simulink model "MyPTControl_RTW"  (Simulink 7.5)
settings: Solver=ode1  SolverMode=SingleTasking  StartTime=0.0  StopTime=inf  FixedStep=0.0002  RelTol=1e-3
PreLoadFcn:
  | vehicle = 'Car'; if ~length(which('cmcmd')), cmenv; end
  | MyPTControl_RTW_bus
InitFcn:
  | vehicle = 'Car'; if ~length(which('cmcmd')), cmenv; end
  | MyPTControl_RTW_bus
undefined symbols (not defined in the file or in its folder): EngineOut_Load, EngineOut_set_ISC, Ignition, ISGOut_Load, OperationState
libraries: simulink x11
Description:
  | CarMaker Real-Time Target (generic)
settings Model: Creator=ml  LastModifiedBy=ml
settings DebuggingCC: SolverPrmCheckMsg=none
settings HardwareCC: TargetHWDeviceType=32-bit Generic  ProdEqTarget=off
settings RTWCC: SystemTargetFile=CarMaker.tlc  TemplateMakefile=CarMaker_unix.tmf  Description=CarMaker Real-Time Target (32-bit)  ProcessScript=CarMaker_make_rtw_hook
settings CodeAppCC: MaxIdLength=63
settings STFCustomTargetCC: ModelReferenceCompliant=off  GeneratePreprocessorConditionals=Disable all  SystemTargetFile=CarMaker.tlc
settings GRTTargetCC: ModelReferenceCompliant=off  ParMdlRefBuildCompliant=off  CompOptLevelCompliant=off  MatFileLogging=off  ExtModeMexFile=noextcomm
settings CustomProperty: DataType=string  Value=..
settings EnumStrPairs: String=Car

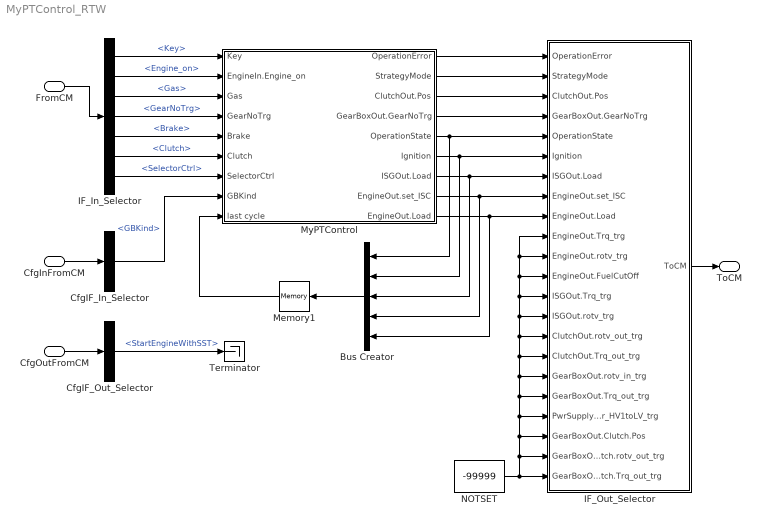
== system MyPTControl_RTW ==
  FromCM : Inport  UseBusObject=on
      settings: BusObject=cmPTControlIn
  CfgInFromCM : Inport  Port=2  UseBusObject=on
      settings: BusObject=cmPTControlCfgIn
  CfgOutFromCM : Inport  Port=3  UseBusObject=on
      settings: BusObject=cmPTControlCfgOut
  Bus Creator : BusCreator  Inputs=5
  CfgIF_In_Selector : BusSelector  OutputSignals=GearBox.GBKind
  CfgIF_Out_Selector : BusSelector  OutputSignals=StartEngineWithSST
  IF_In_Selector : BusSelector  OutputSignals=Key,EngineIn.Engine_on,Gas,GearNoTrg,Brake,Clutch,SelectorCtrl
  IF_Out_Selector : Subsystem
      settings: OpenFcn=cmSignalSelect('SignalSelection_CB',gcb)
      mask Type: Signal Selection
      mask Description: Signal Selection Block
  Memory1 : Memory
  MyPTControl : Subsystem
  NOTSET : Constant  Value=-99999  OutDataType=sfix(16)  OutScaling=2^0
  Terminator : Terminator
  ToCM : Outport  UseBusObject=on
      settings: BusObject=cmPTControlOut
  wires:
  FromCM/1 -> IF_In_Selector/1
  IF_Out_Selector/1(ToCM) -> ToCM/1
  Bus Creator/1 -> Memory1/1
  Memory1/1 -> MyPTControl/9(last cycle)
  MyPTControl/5(OperationState) -> Bus Creator/1, IF_Out_Selector/5(OperationState)
  MyPTControl/6(Ignition) -> Bus Creator/2, IF_Out_Selector/6(Ignition)
  MyPTControl/7(ISGOut.Load) -> Bus Creator/3, IF_Out_Selector/7(ISGOut.Load)
  MyPTControl/8(EngineOut.set_ISC) -> Bus Creator/4, IF_Out_Selector/8(EngineOut.set_ISC)
  MyPTControl/9(EngineOut.Load) -> Bus Creator/5, IF_Out_Selector/9(EngineOut.Load)
  MyPTControl/1(OperationError) -> IF_Out_Selector/1(OperationError)
  MyPTControl/2(StrategyMode) -> IF_Out_Selector/2(StrategyMode)
  MyPTControl/3(ClutchOut.Pos) -> IF_Out_Selector/3(ClutchOut.Pos)
  MyPTControl/4(GearBoxOut.GearNoTrg) -> IF_Out_Selector/4(GearBoxOut.GearNoTrg)
  NOTSET/1 -> IF_Out_Selector/21(GearBoxOut.Clutch.rotv_out_trg), IF_Out_Selector/22(GearBoxOut.Clutch.Trq_out_trg), IF_Out_Selector/20(GearBoxOut.Clutch.Pos), IF_Out_Selector/19(PwrSupplyOut.Pwr_HV1toLV_trg), IF_Out_Selector/11(EngineOut.rotv_trg), IF_Out_Selector/10(EngineOut.Trq_trg), IF_Out_Selector/12(EngineOut.FuelCutOff), IF_Out_Selector/13(ISGOut.Trq_trg), IF_Out_Selector/14(ISGOut.rotv_trg), IF_Out_Selector/15(ClutchOut.rotv_out_trg), IF_Out_Selector/16(ClutchOut.Trq_out_trg), IF_Out_Selector/17(GearBoxOut.rotv_in_trg), IF_Out_Selector/18(GearBoxOut.Trq_out_trg)
  IF_In_Selector/1 -> MyPTControl/1(Key)  "<Key>"
  IF_In_Selector/2 -> MyPTControl/2(EngineIn.Engine_on)  "<Engine_on>"
  IF_In_Selector/3 -> MyPTControl/3(Gas)  "<Gas>"
  IF_In_Selector/4 -> MyPTControl/4(GearNoTrg)  "<GearNoTrg>"
  IF_In_Selector/5 -> MyPTControl/5(Brake)  "<Brake>"
  IF_In_Selector/6 -> MyPTControl/6(Clutch)  "<Clutch>"
  IF_In_Selector/7 -> MyPTControl/7(SelectorCtrl)  "<SelectorCtrl>"
  CfgInFromCM/1 -> CfgIF_In_Selector/1
  CfgOutFromCM/1 -> CfgIF_Out_Selector/1
  CfgIF_In_Selector/1 -> MyPTControl/8(GBKind)  "<GBKind>"
  CfgIF_Out_Selector/1 -> Terminator/1  "<StartEngineWithSST>"

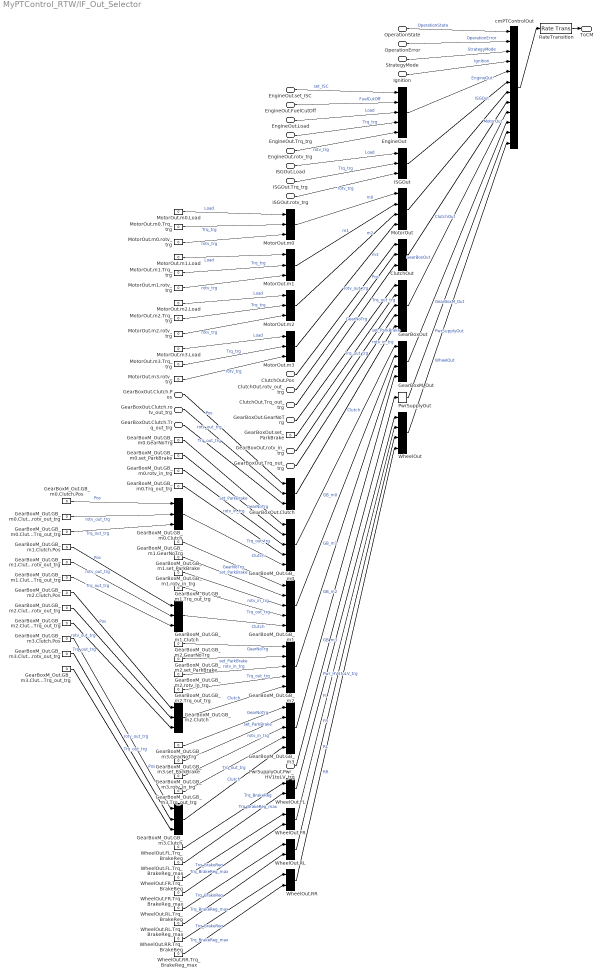
== system MyPTControl_RTW/IF_Out_Selector ==
  OperationError : Inport
  StrategyMode : Inport  Port=2
  ClutchOut.Pos : Inport  Port=3
  GearBoxOut.GearNoTrg : Inport  Port=4
  OperationState : Inport  Port=5
  Ignition : Inport  Port=6
  ISGOut.Load : Inport  Port=7
  EngineOut.set_ISC : Inport  Port=8
  EngineOut.Load : Inport  Port=9
  EngineOut.Trq_trg : Inport  Port=10
  EngineOut.rotv_trg : Inport  Port=11
  EngineOut.FuelCutOff : Inport  Port=12
  ISGOut.Trq_trg : Inport  Port=13
  ISGOut.rotv_trg : Inport  Port=14
  ClutchOut.rotv_out_trg : Inport  Port=15
  ClutchOut.Trq_out_trg : Inport  Port=16
  GearBoxOut.rotv_in_trg : Inport  Port=17
  GearBoxOut.Trq_out_trg : Inport  Port=18
  PwrSupplyOut.Pwr_HV1toLV_trg : Inport  Port=19
  GearBoxOut.Clutch.Pos : Inport  Port=20
  GearBoxOut.Clutch.rotv_out_trg : Inport  Port=21
  GearBoxOut.Clutch.Trq_out_trg : Inport  Port=22
  ClutchOut : BusCreator  Inputs=3
  EngineOut : BusCreator  Inputs=5
  GearBoxM_Out : BusCreator
  GearBoxM_Out.GB_m{0..3} (4 alike) : BusCreator  Inputs=5
  GearBoxM_Out.GB_m0.Clutch : BusCreator  Inputs=3
  GearBoxM_Out.GB_m0.Clutch.Pos : Constant  Value=0
  GearBoxM_Out.GB_m0.Clutch.Trq_out_trg : Constant  Value=0
  GearBoxM_Out.GB_m0.Clutch.rotv_out_trg : Constant  Value=0
  GearBoxM_Out.GB_m0.GearNoTrg : Constant  Value=0
  GearBoxM_Out.GB_m0.Trq_out_trg : Constant  Value=0
  GearBoxM_Out.GB_m0.rotv_in_trg : Constant  Value=0
  GearBoxM_Out.GB_m0.set_ParkBrake : Constant  Value=0
  GearBoxM_Out.GB_m1.Clutch : BusCreator  Inputs=3
  GearBoxM_Out.GB_m1.Clutch.Pos : Constant  Value=0
  GearBoxM_Out.GB_m1.Clutch.Trq_out_trg : Constant  Value=0
  GearBoxM_Out.GB_m1.Clutch.rotv_out_trg : Constant  Value=0
  GearBoxM_Out.GB_m1.GearNoTrg : Constant  Value=0
  GearBoxM_Out.GB_m1.Trq_out_trg : Constant  Value=0
  GearBoxM_Out.GB_m1.rotv_in_trg : Constant  Value=0
  GearBoxM_Out.GB_m1.set_ParkBrake : Constant  Value=0
  GearBoxM_Out.GB_m2.Clutch : BusCreator  Inputs=3
  GearBoxM_Out.GB_m2.Clutch.Pos : Constant  Value=0
  GearBoxM_Out.GB_m2.Clutch.Trq_out_trg : Constant  Value=0
  GearBoxM_Out.GB_m2.Clutch.rotv_out_trg : Constant  Value=0
  GearBoxM_Out.GB_m2.GearNoTrg : Constant  Value=0
  GearBoxM_Out.GB_m2.Trq_out_trg : Constant  Value=0
  GearBoxM_Out.GB_m2.rotv_in_trg : Constant  Value=0
  GearBoxM_Out.GB_m2.set_ParkBrake : Constant  Value=0
  GearBoxM_Out.GB_m3.Clutch : BusCreator  Inputs=3
  GearBoxM_Out.GB_m3.Clutch.Pos : Constant  Value=0
  GearBoxM_Out.GB_m3.Clutch.Trq_out_trg : Constant  Value=0
  GearBoxM_Out.GB_m3.Clutch.rotv_out_trg : Constant  Value=0
  GearBoxM_Out.GB_m3.GearNoTrg : Constant  Value=0
  GearBoxM_Out.GB_m3.Trq_out_trg : Constant  Value=0
  GearBoxM_Out.GB_m3.rotv_in_trg : Constant  Value=0
  GearBoxM_Out.GB_m3.set_ParkBrake : Constant  Value=0
  GearBoxOut : BusCreator  Inputs=5
  GearBoxOut.Clutch : BusCreator  Inputs=3
  GearBoxOut.set_ParkBrake : Constant  Value=0
  ISGOut : BusCreator  Inputs=3
  MotorOut : BusCreator
  MotorOut.m{0..3} (4 alike) : BusCreator  Inputs=3
  MotorOut.m0.Load : Constant  Value=0
  MotorOut.m0.Trq_trg : Constant  Value=0
  MotorOut.m0.rotv_trg : Constant  Value=0
  MotorOut.m1.Load : Constant  Value=0
  MotorOut.m1.Trq_trg : Constant  Value=0
  MotorOut.m1.rotv_trg : Constant  Value=0
  MotorOut.m2.Load : Constant  Value=0
  MotorOut.m2.Trq_trg : Constant  Value=0
  MotorOut.m2.rotv_trg : Constant  Value=0
  MotorOut.m3.Load : Constant  Value=0
  MotorOut.m3.Trq_trg : Constant  Value=0
  MotorOut.m3.rotv_trg : Constant  Value=0
  PwrSupplyOut : BusCreator  Inputs=1
  RateTransition : RateTransition  OutPortSampleTime=str2num(get_param(gcs,'FixedStep'))
  WheelOut : BusCreator
  WheelOut.FL : BusCreator  Inputs=2
  WheelOut.FL.Trq_BrakeReg : Constant  Value=0
  WheelOut.FL.Trq_BrakeReg_max : Constant  Value=0
  WheelOut.FR : BusCreator  Inputs=2
  WheelOut.FR.Trq_BrakeReg : Constant  Value=0
  WheelOut.FR.Trq_BrakeReg_max : Constant  Value=0
  WheelOut.RL : BusCreator  Inputs=2
  WheelOut.RL.Trq_BrakeReg : Constant  Value=0
  WheelOut.RL.Trq_BrakeReg_max : Constant  Value=0
  WheelOut.RR : BusCreator  Inputs=2
  WheelOut.RR.Trq_BrakeReg : Constant  Value=0
  WheelOut.RR.Trq_BrakeReg_max : Constant  Value=0
  cmPTControlOut : BusCreator  Inputs=12
  ToCM : Outport
  wires:
  RateTransition/1 -> ToCM/1
  cmPTControlOut/1 -> RateTransition/1
  EngineOut/1 -> cmPTControlOut/5  "EngineOut"
  ISGOut/1 -> cmPTControlOut/6  "ISGOut"
  MotorOut/1 -> cmPTControlOut/7  "MotorOut"
  MotorOut.m0/1 -> MotorOut/1  "m0"
  MotorOut.m0.Load/1 -> MotorOut.m0/1  "Load"
  MotorOut.m0.Trq_trg/1 -> MotorOut.m0/2  "Trq_trg"
  MotorOut.m0.rotv_trg/1 -> MotorOut.m0/3  "rotv_trg"
  MotorOut.m1/1 -> MotorOut/2  "m1"
  MotorOut.m1.Load/1 -> MotorOut.m1/1  "Load"
  MotorOut.m1.Trq_trg/1 -> MotorOut.m1/2  "Trq_trg"
  MotorOut.m1.rotv_trg/1 -> MotorOut.m1/3  "rotv_trg"
  MotorOut.m2/1 -> MotorOut/3  "m2"
  MotorOut.m2.Load/1 -> MotorOut.m2/1  "Load"
  MotorOut.m2.Trq_trg/1 -> MotorOut.m2/2  "Trq_trg"
  MotorOut.m2.rotv_trg/1 -> MotorOut.m2/3  "rotv_trg"
  MotorOut.m3/1 -> MotorOut/4  "m3"
  MotorOut.m3.Load/1 -> MotorOut.m3/1  "Load"
  MotorOut.m3.Trq_trg/1 -> MotorOut.m3/2  "Trq_trg"
  MotorOut.m3.rotv_trg/1 -> MotorOut.m3/3  "rotv_trg"
  ClutchOut/1 -> cmPTControlOut/8  "ClutchOut"
  GearBoxOut/1 -> cmPTControlOut/9  "GearBoxOut"
  GearBoxOut.set_ParkBrake/1 -> GearBoxOut/2  "set_ParkBrake"
  GearBoxOut.Clutch/1 -> GearBoxOut/5  "Clutch"
  GearBoxM_Out/1 -> cmPTControlOut/10  "GearBoxM_Out"
  GearBoxM_Out.GB_m0/1 -> GearBoxM_Out/1  "GB_m0"
  GearBoxM_Out.GB_m0.GearNoTrg/1 -> GearBoxM_Out.GB_m0/1  "GearNoTrg"
  GearBoxM_Out.GB_m0.set_ParkBrake/1 -> GearBoxM_Out.GB_m0/2  "set_ParkBrake"
  GearBoxM_Out.GB_m0.rotv_in_trg/1 -> GearBoxM_Out.GB_m0/3  "rotv_in_trg"
  GearBoxM_Out.GB_m0.Trq_out_trg/1 -> GearBoxM_Out.GB_m0/4  "Trq_out_trg"
  GearBoxM_Out.GB_m0.Clutch/1 -> GearBoxM_Out.GB_m0/5  "Clutch"
  GearBoxM_Out.GB_m0.Clutch.Pos/1 -> GearBoxM_Out.GB_m0.Clutch/1  "Pos"
  GearBoxM_Out.GB_m0.Clutch.rotv_out_trg/1 -> GearBoxM_Out.GB_m0.Clutch/2  "rotv_out_trg"
  GearBoxM_Out.GB_m0.Clutch.Trq_out_trg/1 -> GearBoxM_Out.GB_m0.Clutch/3  "Trq_out_trg"
  GearBoxM_Out.GB_m1/1 -> GearBoxM_Out/2  "GB_m1"
  GearBoxM_Out.GB_m1.GearNoTrg/1 -> GearBoxM_Out.GB_m1/1  "GearNoTrg"
  GearBoxM_Out.GB_m1.set_ParkBrake/1 -> GearBoxM_Out.GB_m1/2  "set_ParkBrake"
  GearBoxM_Out.GB_m1.rotv_in_trg/1 -> GearBoxM_Out.GB_m1/3  "rotv_in_trg"
  GearBoxM_Out.GB_m1.Trq_out_trg/1 -> GearBoxM_Out.GB_m1/4  "Trq_out_trg"
  GearBoxM_Out.GB_m1.Clutch/1 -> GearBoxM_Out.GB_m1/5  "Clutch"
  GearBoxM_Out.GB_m1.Clutch.Pos/1 -> GearBoxM_Out.GB_m1.Clutch/1  "Pos"
  GearBoxM_Out.GB_m1.Clutch.rotv_out_trg/1 -> GearBoxM_Out.GB_m1.Clutch/2  "rotv_out_trg"
  GearBoxM_Out.GB_m1.Clutch.Trq_out_trg/1 -> GearBoxM_Out.GB_m1.Clutch/3  "Trq_out_trg"
  GearBoxM_Out.GB_m2/1 -> GearBoxM_Out/3  "GB_m2"
  GearBoxM_Out.GB_m2.GearNoTrg/1 -> GearBoxM_Out.GB_m2/1  "GearNoTrg"
  GearBoxM_Out.GB_m2.set_ParkBrake/1 -> GearBoxM_Out.GB_m2/2  "set_ParkBrake"
  GearBoxM_Out.GB_m2.rotv_in_trg/1 -> GearBoxM_Out.GB_m2/3  "rotv_in_trg"
  GearBoxM_Out.GB_m2.Trq_out_trg/1 -> GearBoxM_Out.GB_m2/4  "Trq_out_trg"
  GearBoxM_Out.GB_m2.Clutch/1 -> GearBoxM_Out.GB_m2/5  "Clutch"
  GearBoxM_Out.GB_m2.Clutch.Pos/1 -> GearBoxM_Out.GB_m2.Clutch/1  "Pos"
  GearBoxM_Out.GB_m2.Clutch.rotv_out_trg/1 -> GearBoxM_Out.GB_m2.Clutch/2  "rotv_out_trg"
  GearBoxM_Out.GB_m2.Clutch.Trq_out_trg/1 -> GearBoxM_Out.GB_m2.Clutch/3  "Trq_out_trg"
  GearBoxM_Out.GB_m3/1 -> GearBoxM_Out/4  "GB_m3"
  GearBoxM_Out.GB_m3.GearNoTrg/1 -> GearBoxM_Out.GB_m3/1  "GearNoTrg"
  GearBoxM_Out.GB_m3.set_ParkBrake/1 -> GearBoxM_Out.GB_m3/2  "set_ParkBrake"
  GearBoxM_Out.GB_m3.rotv_in_trg/1 -> GearBoxM_Out.GB_m3/3  "rotv_in_trg"
  GearBoxM_Out.GB_m3.Trq_out_trg/1 -> GearBoxM_Out.GB_m3/4  "Trq_out_trg"
  GearBoxM_Out.GB_m3.Clutch/1 -> GearBoxM_Out.GB_m3/5  "Clutch"
  GearBoxM_Out.GB_m3.Clutch.Pos/1 -> GearBoxM_Out.GB_m3.Clutch/1  "Pos"
  GearBoxM_Out.GB_m3.Clutch.rotv_out_trg/1 -> GearBoxM_Out.GB_m3.Clutch/2  "rotv_out_trg"
  GearBoxM_Out.GB_m3.Clutch.Trq_out_trg/1 -> GearBoxM_Out.GB_m3.Clutch/3  "Trq_out_trg"
  PwrSupplyOut/1 -> cmPTControlOut/11  "PwrSupplyOut"
  WheelOut/1 -> cmPTControlOut/12  "WheelOut"
  WheelOut.FL/1 -> WheelOut/1  "FL"
  WheelOut.FL.Trq_BrakeReg/1 -> WheelOut.FL/1  "Trq_BrakeReg"
  WheelOut.FL.Trq_BrakeReg_max/1 -> WheelOut.FL/2  "Trq_BrakeReg_max"
  WheelOut.FR/1 -> WheelOut/2  "FR"
  WheelOut.FR.Trq_BrakeReg/1 -> WheelOut.FR/1  "Trq_BrakeReg"
  WheelOut.FR.Trq_BrakeReg_max/1 -> WheelOut.FR/2  "Trq_BrakeReg_max"
  WheelOut.RL/1 -> WheelOut/3  "RL"
  WheelOut.RL.Trq_BrakeReg/1 -> WheelOut.RL/1  "Trq_BrakeReg"
  WheelOut.RL.Trq_BrakeReg_max/1 -> WheelOut.RL/2  "Trq_BrakeReg_max"
  WheelOut.RR/1 -> WheelOut/4  "RR"
  WheelOut.RR.Trq_BrakeReg/1 -> WheelOut.RR/1  "Trq_BrakeReg"
  WheelOut.RR.Trq_BrakeReg_max/1 -> WheelOut.RR/2  "Trq_BrakeReg_max"
  OperationError/1 -> cmPTControlOut/2  "OperationError"
  StrategyMode/1 -> cmPTControlOut/3  "StrategyMode"
  ClutchOut.Pos/1 -> ClutchOut/1  "Pos"
  GearBoxOut.GearNoTrg/1 -> GearBoxOut/1  "GearNoTrg"
  OperationState/1 -> cmPTControlOut/1  "OperationState"
  Ignition/1 -> cmPTControlOut/4  "Ignition"
  ISGOut.Load/1 -> ISGOut/1  "Load"
  EngineOut.set_ISC/1 -> EngineOut/1  "set_ISC"
  EngineOut.Load/1 -> EngineOut/3  "Load"
  EngineOut.Trq_trg/1 -> EngineOut/4  "Trq_trg"
  EngineOut.rotv_trg/1 -> EngineOut/5  "rotv_trg"
  EngineOut.FuelCutOff/1 -> EngineOut/2  "FuelCutOff"
  ISGOut.Trq_trg/1 -> ISGOut/2  "Trq_trg"
  ISGOut.rotv_trg/1 -> ISGOut/3  "rotv_trg"
  ClutchOut.rotv_out_trg/1 -> ClutchOut/2  "rotv_out_trg"
  ClutchOut.Trq_out_trg/1 -> ClutchOut/3  "Trq_out_trg"
  GearBoxOut.rotv_in_trg/1 -> GearBoxOut/3  "rotv_in_trg"
  GearBoxOut.Trq_out_trg/1 -> GearBoxOut/4  "Trq_out_trg"
  PwrSupplyOut.Pwr_HV1toLV_trg/1 -> PwrSupplyOut/1  "Pwr_HV1toLV_trg"
  GearBoxOut.Clutch.Pos/1 -> GearBoxOut.Clutch/1  "Pos"
  GearBoxOut.Clutch.rotv_out_trg/1 -> GearBoxOut.Clutch/2  "rotv_out_trg"
  GearBoxOut.Clutch.Trq_out_trg/1 -> GearBoxOut.Clutch/3  "Trq_out_trg"

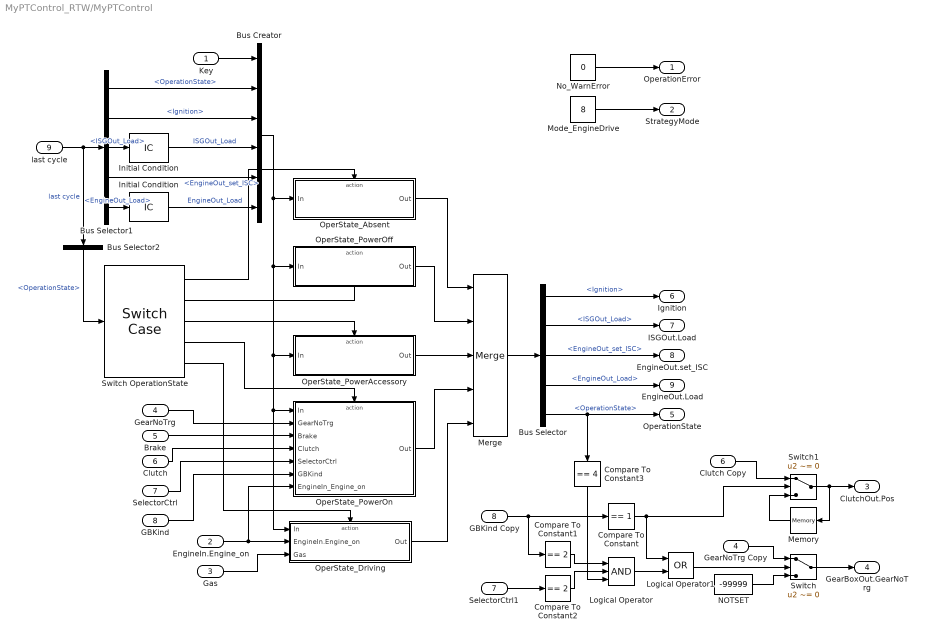
== system MyPTControl_RTW/MyPTControl ==
  Key : Inport  OutDataType=sfix(16)  OutScaling=2^0
  EngineIn.Engine_on : Inport  Port=2  OutDataType=sfix(16)  OutScaling=2^0
  Gas : Inport  Port=3  OutDataType=sfix(16)  OutScaling=2^0
  GearNoTrg : Inport  Port=4  OutDataType=sfix(16)  OutScaling=2^0
  Brake : Inport  Port=5  OutDataType=sfix(16)  OutScaling=2^0
  Clutch : Inport  Port=6  OutDataType=sfix(16)  OutScaling=2^0
  SelectorCtrl : Inport  Port=7  OutDataType=sfix(16)  OutScaling=2^0
  GBKind : Inport  Port=8  OutDataType=sfix(16)  OutScaling=2^0
  last cycle : Inport  Port=9  OutDataType=sfix(16)  OutScaling=2^0
  Bus Creator : BusCreator  Inputs=6
  Bus Selector : BusSelector  OutputSignals=Ignition,ISGOut_Load,EngineOut_set_ISC,EngineOut_Load,OperationState
  Bus Selector1 : BusSelector  OutputSignals=OperationState,Ignition,ISGOut_Load,EngineOut_set_ISC,EngineOut_Load
  Bus Selector2 : BusSelector  OutputSignals=OperationState
  Clutch Copy : InportShadow  Port=6  OutDataType=sfix(16)  OutScaling=2^0
  Compare To Constant : simulink/Logic and Bit Operations/Compare To Constant  SystemSampleTime=-1  relop===  const=1  LogicOutDataTypeMode=uint8  ZeroCross=off
  Compare To Constant1 : simulink/Logic and Bit Operations/Compare To Constant  SystemSampleTime=-1  relop===  const=2  LogicOutDataTypeMode=uint8  ZeroCross=off
  Compare To Constant2 : simulink/Logic and Bit Operations/Compare To Constant  SystemSampleTime=-1  relop===  const=2  LogicOutDataTypeMode=uint8  ZeroCross=off
  Compare To Constant3 : simulink/Logic and Bit Operations/Compare To Constant  SystemSampleTime=-1  relop===  const=4  LogicOutDataTypeMode=uint8  ZeroCross=off
  GBKind Copy : InportShadow  Port=8  OutDataType=sfix(16)  OutScaling=2^0
  GearNoTrg Copy : InportShadow  Port=4  OutDataType=sfix(16)  OutScaling=2^0
  Initial Condition : InitialCondition  Value=-99999
  "Initial Condition " : InitialCondition  Value=-99999
  Logical Operator : Logic  Inputs=3  AllPortsSameDT=off  OutDataTypeMode=boolean  OutDataTypeStr=boolean
  Logical Operator1 : Logic  Operator=OR  AllPortsSameDT=off  OutDataTypeMode=boolean  OutDataTypeStr=boolean
  Memory : Memory
  Merge : Merge  Inputs=5
  Mode_EngineDrive : Constant  Value=8  OutDataType=sfix(16)  OutScaling=2^0
  NOTSET : Constant  Value=-99999  OutDataType=sfix(16)  OutScaling=2^0
  No_WarnError : Constant  Value=0  OutDataType=sfix(16)  OutScaling=2^0
  OperState_Absent : Subsystem  TreatAsAtomicUnit=on
  OperState_Driving : Subsystem  TreatAsAtomicUnit=on
  OperState_PowerAccessory : Subsystem  TreatAsAtomicUnit=on
  OperState_PowerOff : Subsystem  TreatAsAtomicUnit=on
  OperState_PowerOn : Subsystem  TreatAsAtomicUnit=on
  SelectorCtrl1 : InportShadow  Port=7  OutDataType=sfix(16)  OutScaling=2^0
  Switch : Switch  Criteria=u2 ~= 0  OutDataType=sfix(16)  OutScaling=2^0
  Switch OperationState : SwitchCase  CaseConditions={0 1 2 3}
  Switch1 : Switch  Criteria=u2 ~= 0  OutDataType=sfix(16)  OutScaling=2^0
  OperationError : Outport  OutDataType=sfix(16)  OutScaling=2^0
  StrategyMode : Outport  Port=2  OutDataType=sfix(16)  OutScaling=2^0
  ClutchOut.Pos : Outport  Port=3  OutDataType=sfix(16)  OutScaling=2^0
  GearBoxOut.GearNoTrg : Outport  Port=4  OutDataType=sfix(16)  OutScaling=2^0
  OperationState : Outport  Port=5  OutDataType=sfix(16)  OutScaling=2^0
  Ignition : Outport  Port=6  OutDataType=sfix(16)  OutScaling=2^0
  ISGOut.Load : Outport  Port=7  OutDataType=sfix(16)  OutScaling=2^0
  EngineOut.set_ISC : Outport  Port=8  OutDataType=sfix(16)  OutScaling=2^0
  EngineOut.Load : Outport  Port=9  OutDataType=sfix(16)  OutScaling=2^0
  wires:
  No_WarnError/1 -> OperationError/1
  Mode_EngineDrive/1 -> StrategyMode/1
  Switch OperationState/3 -> OperState_PowerAccessory/Action
  Bus Selector/1 -> Ignition/1  "<Ignition>"
  Bus Selector/5 -> OperationState/1, Compare To Constant3/1  "<OperationState>"
  EngineIn.Engine_on/1 -> OperState_PowerOn/7(EngineIn_Engine_on), OperState_Driving/2(EngineIn.Engine_on)
  last cycle/1 -> Bus Selector2/1, Bus Selector1/1  "last cycle"
  Bus Selector2/1 -> Switch OperationState/1  "<OperationState>"
  Key/1 -> Bus Creator/1
  Bus Creator/1 -> OperState_Absent/1(In), OperState_PowerOff/1(In), OperState_PowerAccessory/1(In), OperState_PowerOn/1(In), OperState_Driving/1(In)
  Bus Selector/2 -> ISGOut.Load/1  "<ISGOut_Load>"
  Bus Selector/3 -> EngineOut.set_ISC/1  "<EngineOut_set_ISC>"
  Bus Selector/4 -> EngineOut.Load/1  "<EngineOut_Load>"
  GearNoTrg/1 -> OperState_PowerOn/2(GearNoTrg)
  Brake/1 -> OperState_PowerOn/3(Brake)
  Clutch/1 -> OperState_PowerOn/4(Clutch)
  SelectorCtrl/1 -> OperState_PowerOn/5(SelectorCtrl)
  GBKind/1 -> OperState_PowerOn/6(GBKind)
  Gas/1 -> OperState_Driving/3(Gas)
  Switch OperationState/2 -> OperState_PowerOff/Action
  Switch OperationState/4 -> OperState_PowerOn/Action
  Switch OperationState/5 -> OperState_Driving/Action
  Switch OperationState/1 -> OperState_Absent/Action
  Bus Selector1/1 -> Bus Creator/2  "<OperationState>"
  Bus Selector1/2 -> Bus Creator/3  "<Ignition>"
  Bus Selector1/3 -> Initial Condition/1  "<ISGOut_Load>"
  Bus Selector1/4 -> Bus Creator/5  "<EngineOut_set_ISC>"
  Bus Selector1/5 -> "Initial Condition "/1  "<EngineOut_Load>"
  OperState_PowerOff/1(Out) -> Merge/2
  OperState_PowerAccessory/1(Out) -> Merge/3
  OperState_PowerOn/1(Out) -> Merge/4
  OperState_Driving/1(Out) -> Merge/5
  Merge/1 -> Bus Selector/1
  Compare To Constant1/1 -> Logical Operator/1
  Compare To Constant2/1 -> Logical Operator/2
  Logical Operator/1 -> Logical Operator1/2
  Compare To Constant/1 -> Logical Operator1/1, Switch1/2
  Logical Operator1/1 -> Switch/2
  NOTSET/1 -> Switch/3
  GearNoTrg Copy/1 -> Switch/1
  Switch/1 -> GearBoxOut.GearNoTrg/1
  Switch1/1 -> ClutchOut.Pos/1, Memory/1
  Clutch Copy/1 -> Switch1/1
  Memory/1 -> Switch1/3
  "Initial Condition "/1 -> Bus Creator/6  "EngineOut_Load"
  Initial Condition/1 -> Bus Creator/4  "ISGOut_Load"
  OperState_Absent/1(Out) -> Merge/1
  SelectorCtrl1/1 -> Compare To Constant2/1
  GBKind Copy/1 -> Compare To Constant/1, Compare To Constant1/1
  Compare To Constant3/1 -> Logical Operator/3

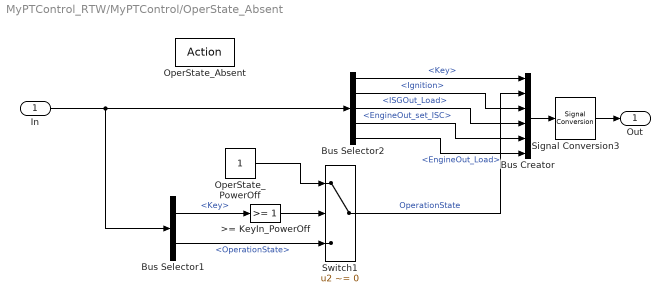
== system MyPTControl_RTW/MyPTControl/OperState_Absent ==
  In : Inport  OutDataType=sfix(16)  OutScaling=2^0
  OperState_Absent : ActionPort  ActionType=case
  >= KeyIn_PowerOff : simulink/Logic and Bit Operations/Compare To Constant  SystemSampleTime=-1  relop=>=  const=1  LogicOutDataTypeMode=uint8  ZeroCross=off
  Bus Creator : BusCreator  Inputs=6
  Bus Selector1 : BusSelector  OutputSignals=Key,OperationState
  Bus Selector2 : BusSelector  OutputSignals=Key,Ignition,ISGOut_Load,EngineOut_set_ISC,EngineOut_Load
  OperState_PowerOff : Constant  OutDataType=sfix(16)  OutScaling=2^0
  Signal Conversion3 : SignalConversion  ConversionOutput=Bus copy
  Switch1 : Switch  Criteria=u2 ~= 0  Threshold=1  OutDataType=sfix(16)  OutScaling=2^0
  Out : Outport  OutDataType=sfix(16)  OutScaling=2^0
  wires:
  In/1 -> Bus Selector1/1, Bus Selector2/1
  Bus Selector1/1 -> >= KeyIn_PowerOff/1  "<Key>"
  OperState_PowerOff/1 -> Switch1/1
  Bus Selector1/2 -> Switch1/3  "<OperationState>"
  Bus Creator/1 -> Signal Conversion3/1
  Signal Conversion3/1 -> Out/1
  Switch1/1 -> Bus Creator/2  "OperationState"
  Bus Selector2/1 -> Bus Creator/1  "<Key>"
  Bus Selector2/2 -> Bus Creator/3  "<Ignition>"
  Bus Selector2/3 -> Bus Creator/4  "<ISGOut_Load>"
  Bus Selector2/4 -> Bus Creator/5  "<EngineOut_set_ISC>"
  Bus Selector2/5 -> Bus Creator/6  "<EngineOut_Load>"
  >= KeyIn_PowerOff/1 -> Switch1/2

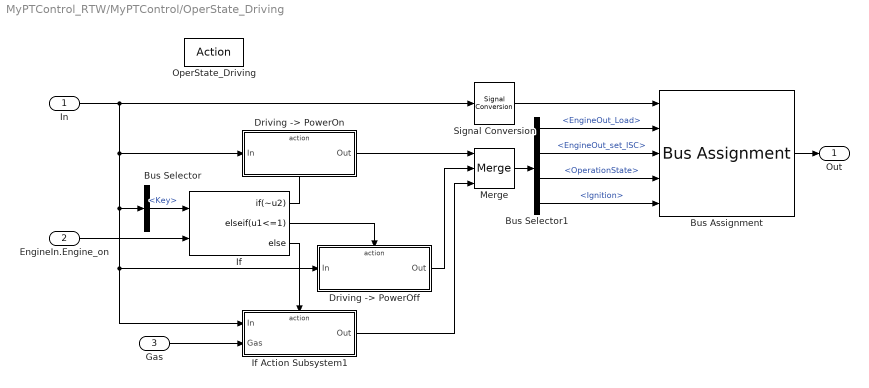
== system MyPTControl_RTW/MyPTControl/OperState_Driving ==
  In : Inport  OutDataType=sfix(16)  OutScaling=2^0
  EngineIn.Engine_on : Inport  Port=2  OutDataType=sfix(16)  OutScaling=2^0
  Gas : Inport  Port=3  OutDataType=sfix(16)  OutScaling=2^0
  OperState_Driving : ActionPort  ActionType=default
  Bus Assignment : BusAssignment  AssignedSignals=EngineOut_Load,EngineOut_set_ISC,OperationState,Ignition
  Bus Selector : BusSelector  OutputSignals=Key
  Bus Selector1 : BusSelector  OutputSignals=EngineOut_Load,EngineOut_set_ISC,OperationState,Ignition
  "Driving -> PowerOff" : Subsystem  TreatAsAtomicUnit=on
  "Driving -> PowerOn" : Subsystem  TreatAsAtomicUnit=on
  If : If  NumInputs=2  IfExpression=~u2  ElseIfExpressions=u1<=1
  If Action Subsystem1 : Subsystem  TreatAsAtomicUnit=on
  Merge : Merge  Inputs=3
  Signal Conversion : SignalConversion  ConversionOutput=Bus copy
  Out : Outport  OutDataType=sfix(16)  OutScaling=2^0
  wires:
  Merge/1 -> Bus Selector1/1
  Bus Assignment/1 -> Out/1
  In/1 -> "Driving -> PowerOn"/1(In), Bus Selector/1, "Driving -> PowerOff"/1(In), If Action Subsystem1/1(In), Signal Conversion/1
  If/3 -> If Action Subsystem1/Action
  If/1 -> "Driving -> PowerOn"/Action
  If/2 -> "Driving -> PowerOff"/Action
  Bus Selector/1 -> If/1  "<Key>"
  EngineIn.Engine_on/1 -> If/2
  If Action Subsystem1/1(Out) -> Merge/3
  "Driving -> PowerOn"/1(Out) -> Merge/1
  Bus Selector1/1 -> Bus Assignment/2  "<EngineOut_Load>"
  Bus Selector1/2 -> Bus Assignment/3  "<EngineOut_set_ISC>"
  Bus Selector1/3 -> Bus Assignment/4  "<OperationState>"
  Bus Selector1/4 -> Bus Assignment/5  "<Ignition>"
  Gas/1 -> If Action Subsystem1/2(Gas)
  "Driving -> PowerOff"/1(Out) -> Merge/2
  Signal Conversion/1 -> Bus Assignment/1

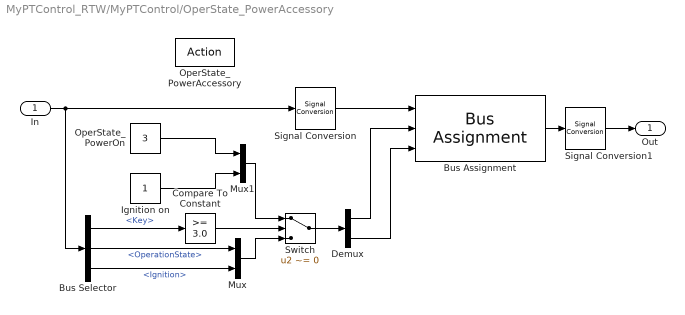
== system MyPTControl_RTW/MyPTControl/OperState_PowerAccessory ==
  In : Inport  OutDataType=sfix(16)  OutScaling=2^0
  OperState_PowerAccessory : ActionPort  ActionType=case
  Bus Assignment : BusAssignment  AssignedSignals=OperationState,Ignition
  Bus Selector : BusSelector  OutputSignals=Key,OperationState,Ignition
  Compare To Constant : simulink/Logic and Bit Operations/Compare To Constant  SystemSampleTime=-1  relop=>=  const=3.0  LogicOutDataTypeMode=uint8  ZeroCross=off
  Demux : Demux  Outputs=2
  Ignition on : Constant  OutDataType=sfix(16)  OutScaling=2^0
  Mux : Mux  Inputs=2
  Mux1 : Mux  Inputs=2
  OperState_PowerOn : Constant  Value=3  OutDataType=sfix(16)  OutScaling=2^0
  Signal Conversion : SignalConversion  ConversionOutput=Bus copy
  Signal Conversion1 : SignalConversion  ConversionOutput=Bus copy
  Switch : Switch  Criteria=u2 ~= 0  Threshold=3  OutDataType=sfix(16)  OutScaling=2^0
  Out : Outport  OutDataType=sfix(16)  OutScaling=2^0
  wires:
  Bus Selector/1 -> Compare To Constant/1  "<Key>"
  Switch/1 -> Demux/1
  Demux/1 -> Bus Assignment/2
  Demux/2 -> Bus Assignment/3
  Bus Selector/2 -> Mux/1  "<OperationState>"
  Bus Selector/3 -> Mux/2  "<Ignition>"
  Mux/1 -> Switch/3
  Mux1/1 -> Switch/1
  Ignition on/1 -> Mux1/2
  Bus Assignment/1 -> Signal Conversion1/1
  In/1 -> Bus Selector/1, Signal Conversion/1
  OperState_PowerOn/1 -> Mux1/1
  Signal Conversion/1 -> Bus Assignment/1
  Signal Conversion1/1 -> Out/1
  Compare To Constant/1 -> Switch/2

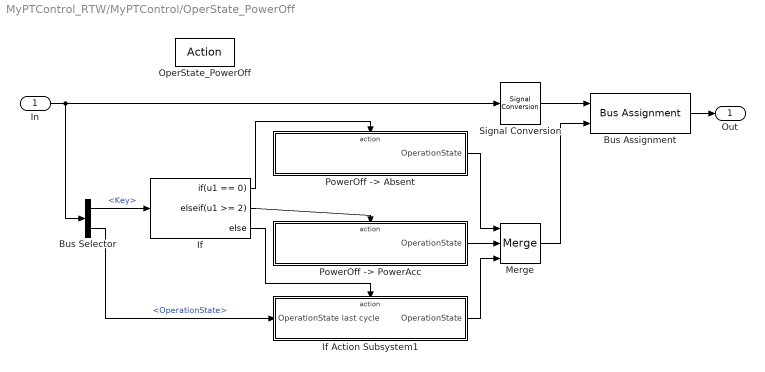
== system MyPTControl_RTW/MyPTControl/OperState_PowerOff ==
  In : Inport  OutDataType=sfix(16)  OutScaling=2^0
  OperState_PowerOff : ActionPort  ActionType=case
  Bus Assignment : BusAssignment  AssignedSignals=OperationState
  Bus Selector : BusSelector  OutputSignals=Key,OperationState
  If : If  IfExpression=u1 == 0  ElseIfExpressions=u1 >= 2
  If Action Subsystem1 : Subsystem  TreatAsAtomicUnit=on
  Merge : Merge  Inputs=3
  "PowerOff -> Absent" : Subsystem  TreatAsAtomicUnit=on
  "PowerOff -> PowerAcc" : Subsystem  TreatAsAtomicUnit=on
  Signal Conversion : SignalConversion  ConversionOutput=Bus copy
  Out : Outport  OutDataType=sfix(16)  OutScaling=2^0
  wires:
  If/1 -> "PowerOff -> Absent"/Action
  Merge/1 -> Bus Assignment/2
  "PowerOff -> Absent"/1(OperationState) -> Merge/1
  Bus Selector/2 -> If Action Subsystem1/1(OperationState last cycle)  "<OperationState>"
  If/2 -> "PowerOff -> PowerAcc"/Action
  "PowerOff -> PowerAcc"/1(OperationState) -> Merge/2
  If Action Subsystem1/1(OperationState) -> Merge/3
  If/3 -> If Action Subsystem1/Action
  Bus Assignment/1 -> Out/1
  In/1 -> Bus Selector/1, Signal Conversion/1
  Bus Selector/1 -> If/1  "<Key>"
  Signal Conversion/1 -> Bus Assignment/1

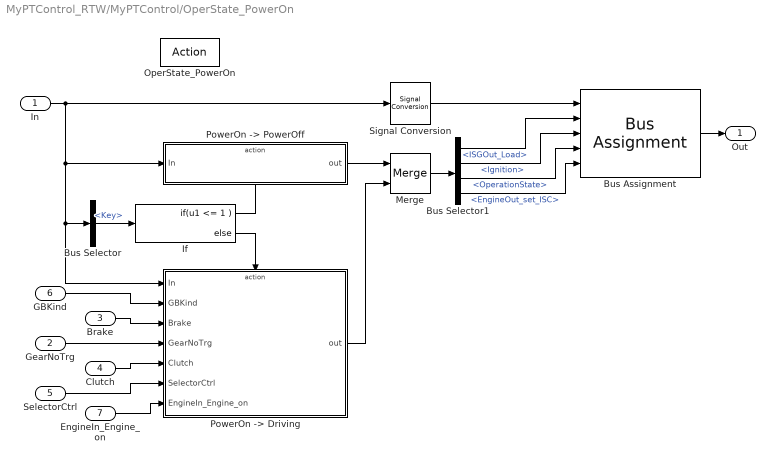
== system MyPTControl_RTW/MyPTControl/OperState_PowerOn ==
  In : Inport  OutDataType=sfix(16)  OutScaling=2^0
  GearNoTrg : Inport  Port=2  OutDataType=sfix(16)  OutScaling=2^0
  Brake : Inport  Port=3  OutDataType=sfix(16)  OutScaling=2^0
  Clutch : Inport  Port=4  OutDataType=sfix(16)  OutScaling=2^0
  SelectorCtrl : Inport  Port=5  OutDataType=sfix(16)  OutScaling=2^0
  GBKind : Inport  Port=6  OutDataType=sfix(16)  OutScaling=2^0
  EngineIn_Engine_on : Inport  Port=7  OutDataType=sfix(16)  OutScaling=2^0
  OperState_PowerOn : ActionPort  ActionType=case
  Bus Assignment : BusAssignment  AssignedSignals=ISGOut_Load,Ignition,OperationState,EngineOut_set_ISC
  Bus Selector : BusSelector  OutputSignals=Key
  Bus Selector1 : BusSelector  OutputSignals=ISGOut_Load,Ignition,OperationState,EngineOut_set_ISC
  If : If  IfExpression=u1 <= 1
  Merge : Merge
  "PowerOn -> Driving" : Subsystem  TreatAsAtomicUnit=on
  "PowerOn -> PowerOff" : Subsystem  TreatAsAtomicUnit=on
  Signal Conversion : SignalConversion  ConversionOutput=Bus copy
  Out : Outport  OutDataType=sfix(16)  OutScaling=2^0
  wires:
  If/1 -> "PowerOn -> PowerOff"/Action
  If/2 -> "PowerOn -> Driving"/Action
  In/1 -> Bus Selector/1, "PowerOn -> Driving"/1(In), "PowerOn -> PowerOff"/1(In), Signal Conversion/1
  Bus Assignment/1 -> Out/1
  Bus Selector/1 -> If/1  "<Key>"
  "PowerOn -> Driving"/1(out) -> Merge/2
  Merge/1 -> Bus Selector1/1
  GBKind/1 -> "PowerOn -> Driving"/2(GBKind)
  Brake/1 -> "PowerOn -> Driving"/3(Brake)
  GearNoTrg/1 -> "PowerOn -> Driving"/4(GearNoTrg)
  Bus Selector1/1 -> Bus Assignment/2  "<ISGOut_Load>"
  Bus Selector1/2 -> Bus Assignment/3  "<Ignition>"
  Bus Selector1/3 -> Bus Assignment/4  "<OperationState>"
  EngineIn_Engine_on/1 -> "PowerOn -> Driving"/7(EngineIn_Engine_on)
  Clutch/1 -> "PowerOn -> Driving"/5(Clutch)
  SelectorCtrl/1 -> "PowerOn -> Driving"/6(SelectorCtrl)
  "PowerOn -> PowerOff"/1(out) -> Merge/1
  Signal Conversion/1 -> Bus Assignment/1
  Bus Selector1/4 -> Bus Assignment/5  "<EngineOut_set_ISC>"

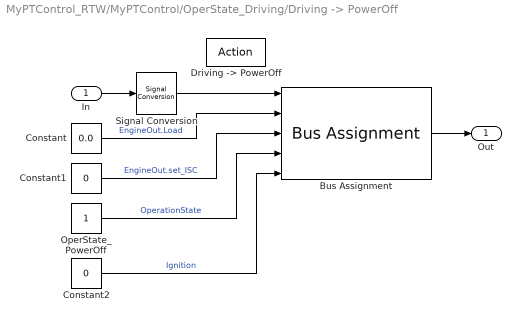
== system MyPTControl_RTW/MyPTControl/OperState_Driving/Driving -> PowerOff ==
  In : Inport  OutDataType=sfix(16)  OutScaling=2^0
  "Driving -> PowerOff" : ActionPort  ActionType=elseif
  Bus Assignment : BusAssignment  AssignedSignals=EngineOut_Load,EngineOut_set_ISC,Ignition,OperationState
  Constant : Constant  Value=0.0  OutDataType=sfix(16)  OutScaling=2^0
  Constant1 : Constant  Value=0  OutDataType=sfix(16)  OutScaling=2^0
  Constant2 : Constant  Value=0  OutDataType=sfix(16)  OutScaling=2^0
  OperState_PowerOff : Constant  OutDataType=sfix(16)  OutScaling=2^0
  Signal Conversion : SignalConversion  ConversionOutput=Bus copy
  Out : Outport  OutDataType=sfix(16)  OutScaling=2^0  InitialOutput=[0, 0, 0, 0, 0, 0]
  wires:
  Constant1/1 -> Bus Assignment/3  "EngineOut.set_ISC"
  OperState_PowerOff/1 -> Bus Assignment/4  "OperationState"
  In/1 -> Signal Conversion/1
  Bus Assignment/1 -> Out/1
  Constant/1 -> Bus Assignment/2  "EngineOut.Load"
  Constant2/1 -> Bus Assignment/5  "Ignition"
  Signal Conversion/1 -> Bus Assignment/1

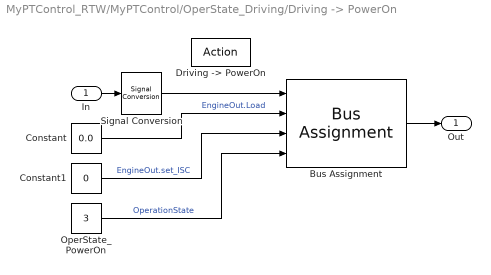
== system MyPTControl_RTW/MyPTControl/OperState_Driving/Driving -> PowerOn ==
  In : Inport  OutDataType=sfix(16)  OutScaling=2^0
  "Driving -> PowerOn" : ActionPort  ActionType=then
  Bus Assignment : BusAssignment  AssignedSignals=EngineOut_Load,EngineOut_set_ISC,OperationState
  Constant : Constant  Value=0.0  OutDataType=sfix(16)  OutScaling=2^0
  Constant1 : Constant  Value=0  OutDataType=sfix(16)  OutScaling=2^0
  OperState_PowerOn : Constant  Value=3  OutDataType=sfix(16)  OutScaling=2^0
  Signal Conversion : SignalConversion  ConversionOutput=Bus copy
  Out : Outport  OutDataType=sfix(16)  OutScaling=2^0  InitialOutput=[0, 0, 0, 0, 0, 0]
  wires:
  Constant/1 -> Bus Assignment/2  "EngineOut.Load"
  Constant1/1 -> Bus Assignment/3  "EngineOut.set_ISC"
  OperState_PowerOn/1 -> Bus Assignment/4  "OperationState"
  In/1 -> Signal Conversion/1
  Bus Assignment/1 -> Out/1
  Signal Conversion/1 -> Bus Assignment/1

== system MyPTControl_RTW/MyPTControl/OperState_Driving/If Action Subsystem1 ==
  In : Inport  OutDataType=sfix(16)  OutScaling=2^0
  Gas : Inport  Port=2  OutDataType=sfix(16)  OutScaling=2^0
  Action Port : ActionPort  ActionType=else
  Bus Assignment : BusAssignment  AssignedSignals=EngineOut_Load
  Gain1 : Gain  ParameterDataType=sfix(16)  ParameterScaling=2^0  OutDataType=sfix(16)  OutScaling=2^0
  Signal Conversion : SignalConversion  ConversionOutput=Bus copy
  Out : Outport  OutDataType=sfix(16)  OutScaling=2^0
  wires:
  Gas/1 -> Gain1/1
  In/1 -> Signal Conversion/1
  Bus Assignment/1 -> Out/1
  Gain1/1 -> Bus Assignment/2  "EngineOut.Load"
  Signal Conversion/1 -> Bus Assignment/1

== system MyPTControl_RTW/MyPTControl/OperState_PowerOff/If Action Subsystem1 ==
  OperationState last cycle : Inport  OutDataType=sfix(16)  OutScaling=2^0
  Action Port : ActionPort  ActionType=else
  OperationState : Outport  OutDataType=sfix(16)  OutScaling=2^0
  wires:
  OperationState last cycle/1 -> OperationState/1

== system MyPTControl_RTW/MyPTControl/OperState_PowerOff/PowerOff -> Absent ==
  "PowerOff -> Absent" : ActionPort  ActionType=then
  OperState_Absent : Constant  Value=0  OutDataType=sfix(16)  OutScaling=2^0
  OperationState : Outport  OutDataType=sfix(16)  OutScaling=2^0  InitialOutput=0
  wires:
  OperState_Absent/1 -> OperationState/1

== system MyPTControl_RTW/MyPTControl/OperState_PowerOff/PowerOff -> PowerAcc ==
  "PowerOff -> PowerAcc" : ActionPort  ActionType=elseif
  OperState_PowerAccesory : Constant  Value=2  OutDataType=sfix(16)  OutScaling=2^0
  OperationState : Outport  OutDataType=sfix(16)  OutScaling=2^0  InitialOutput=2
  wires:
  OperState_PowerAccesory/1 -> OperationState/1

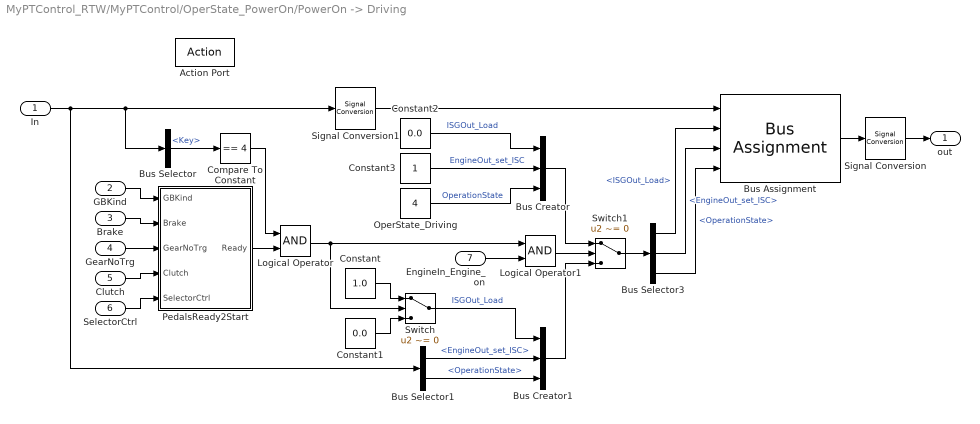
== system MyPTControl_RTW/MyPTControl/OperState_PowerOn/PowerOn -> Driving ==
  In : Inport  OutDataType=sfix(16)  OutScaling=2^0
  GBKind : Inport  Port=2  OutDataType=sfix(16)  OutScaling=2^0
  Brake : Inport  Port=3  OutDataType=sfix(16)  OutScaling=2^0
  GearNoTrg : Inport  Port=4  OutDataType=sfix(16)  OutScaling=2^0
  Clutch : Inport  Port=5  OutDataType=sfix(16)  OutScaling=2^0
  SelectorCtrl : Inport  Port=6  OutDataType=sfix(16)  OutScaling=2^0
  EngineIn_Engine_on : Inport  Port=7  OutDataType=sfix(16)  OutScaling=2^0
  Action Port : ActionPort  ActionType=else
  Bus Assignment : BusAssignment  AssignedSignals=ISGOut_Load,EngineOut_set_ISC,OperationState
  Bus Creator : BusCreator  Inputs=3
  Bus Creator1 : BusCreator  Inputs=3
  Bus Selector : BusSelector  OutputSignals=Key
  Bus Selector1 : BusSelector  OutputSignals=EngineOut_set_ISC,OperationState
  Bus Selector3 : BusSelector  OutputSignals=ISGOut_Load,EngineOut_set_ISC,OperationState
  Compare To Constant : simulink/Logic and Bit Operations/Compare To Constant  SystemSampleTime=-1  relop===  const=4  LogicOutDataTypeMode=uint8  ZeroCross=off
  Constant : Constant  Value=1.0  OutDataType=sfix(16)  OutScaling=2^0
  Constant1 : Constant  Value=0.0  OutDataType=sfix(16)  OutScaling=2^0
  Constant2 : Constant  Value=0.0  OutDataType=sfix(16)  OutScaling=2^0
  Constant3 : Constant  OutDataType=sfix(16)  OutScaling=2^0
  Logical Operator : Logic  AllPortsSameDT=off  OutDataTypeMode=boolean  OutDataTypeStr=boolean
  Logical Operator1 : Logic  AllPortsSameDT=off  OutDataTypeMode=boolean  OutDataTypeStr=boolean
  OperState_Driving : Constant  Value=4  OutDataType=sfix(16)  OutScaling=2^0
  PedalsReady2Start : Subsystem
  Signal Conversion : SignalConversion  ConversionOutput=Bus copy
  Signal Conversion1 : SignalConversion  ConversionOutput=Bus copy
  Switch : Switch  Criteria=u2 ~= 0  OutDataType=sfix(16)  OutScaling=2^0
  Switch1 : Switch  Criteria=u2 ~= 0  OutDataType=sfix(16)  OutScaling=2^0
  out : Outport  OutDataType=sfix(16)  OutScaling=2^0
  wires:
  In/1 -> Bus Selector1/1, Bus Selector/1, Signal Conversion1/1
  Bus Selector/1 -> Compare To Constant/1  "<Key>"
  Compare To Constant/1 -> Logical Operator/1
  PedalsReady2Start/1(Ready) -> Logical Operator/2
  GBKind/1 -> PedalsReady2Start/1(GBKind)
  Brake/1 -> PedalsReady2Start/2(Brake)
  GearNoTrg/1 -> PedalsReady2Start/3(GearNoTrg)
  Clutch/1 -> PedalsReady2Start/4(Clutch)
  SelectorCtrl/1 -> PedalsReady2Start/5(SelectorCtrl)
  Logical Operator/1 -> Switch/2, Logical Operator1/1
  Constant/1 -> Switch/1
  Constant1/1 -> Switch/3
  EngineIn_Engine_on/1 -> Logical Operator1/2
  Bus Selector1/1 -> Bus Creator1/2  "<EngineOut_set_ISC>"
  Bus Selector1/2 -> Bus Creator1/3  "<OperationState>"
  Bus Creator1/1 -> Switch1/3
  Logical Operator1/1 -> Switch1/2
  Switch1/1 -> Bus Selector3/1
  Switch/1 -> Bus Creator1/1  "ISGOut_Load"
  Bus Creator/1 -> Switch1/1
  OperState_Driving/1 -> Bus Creator/3  "OperationState"
  Constant2/1 -> Bus Creator/1  "ISGOut_Load"
  Constant3/1 -> Bus Creator/2  "EngineOut_set_ISC"
  Bus Assignment/1 -> Signal Conversion/1
  Signal Conversion1/1 -> Bus Assignment/1
  Bus Selector3/1 -> Bus Assignment/2  "<ISGOut_Load>"
  Bus Selector3/2 -> Bus Assignment/3  "<EngineOut_set_ISC>"
  Bus Selector3/3 -> Bus Assignment/4  "<OperationState>"
  Signal Conversion/1 -> out/1

== system MyPTControl_RTW/MyPTControl/OperState_PowerOn/PowerOn -> PowerOff ==
  In : Inport  OutDataType=sfix(16)  OutScaling=2^0
  "PowerOn -> PowerOff" : ActionPort  ActionType=then
  Bus Assignment : BusAssignment  AssignedSignals=ISGOut_Load,Ignition,OperationState
  Constant : Constant  Value=0.0  OutDataType=sfix(16)  OutScaling=2^0
  Constant1 : Constant  Value=0  OutDataType=sfix(16)  OutScaling=2^0
  OperState_PowerOff : Constant  OutDataType=sfix(16)  OutScaling=2^0
  Signal Conversion : SignalConversion  ConversionOutput=Bus copy
  out : Outport  OutDataType=sfix(16)  OutScaling=2^0  InitialOutput=[0, 0, 0, 0, 0, 0]
  wires:
  OperState_PowerOff/1 -> Bus Assignment/4  "OperationState"
  Constant/1 -> Bus Assignment/2  "ISGOut_Load"
  Constant1/1 -> Bus Assignment/3  "Ignition"
  In/1 -> Signal Conversion/1
  Bus Assignment/1 -> out/1
  Signal Conversion/1 -> Bus Assignment/1

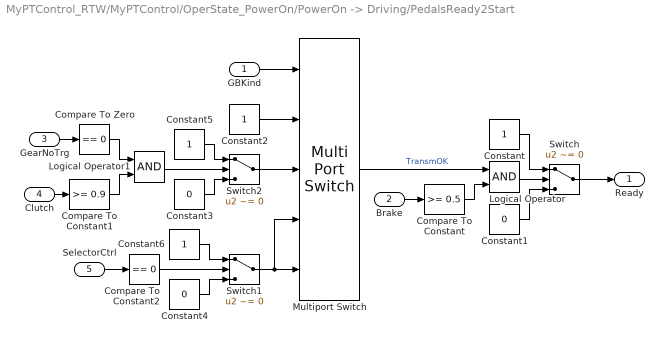
== system MyPTControl_RTW/MyPTControl/OperState_PowerOn/PowerOn -> Driving/PedalsReady2Start ==
  GBKind : Inport  OutDataType=sfix(16)  OutScaling=2^0
  Brake : Inport  Port=2  OutDataType=sfix(16)  OutScaling=2^0
  GearNoTrg : Inport  Port=3  OutDataType=sfix(16)  OutScaling=2^0
  Clutch : Inport  Port=4  OutDataType=sfix(16)  OutScaling=2^0
  SelectorCtrl : Inport  Port=5  OutDataType=sfix(16)  OutScaling=2^0
  Compare To Constant : simulink/Logic and Bit Operations/Compare To Constant  SystemSampleTime=-1  relop=>=  const=0.5  LogicOutDataTypeMode=uint8  ZeroCross=off
  Compare To Constant1 : simulink/Logic and Bit Operations/Compare To Constant  SystemSampleTime=-1  relop=>=  const=0.9  LogicOutDataTypeMode=uint8  ZeroCross=off
  Compare To Constant2 : simulink/Logic and Bit Operations/Compare To Constant  SystemSampleTime=-1  relop===  const=0  LogicOutDataTypeMode=uint8  ZeroCross=off
  Compare To Zero : simulink/Logic and Bit Operations/Compare To Zero  SystemSampleTime=-1  relop===  LogicOutDataTypeMode=uint8  ZeroCross=off
  Constant{,2,5..6} (4 alike) : Constant  OutDataType=sfix(16)  OutScaling=2^0
  Constant1 : Constant  Value=0  OutDataType=sfix(16)  OutScaling=2^0
  Constant3 : Constant  Value=0  OutDataType=sfix(16)  OutScaling=2^0
  Constant4 : Constant  Value=0  OutDataType=sfix(16)  OutScaling=2^0
  Logical Operator : Logic  AllPortsSameDT=off  OutDataTypeMode=boolean  OutDataTypeStr=boolean
  Logical Operator1 : Logic  AllPortsSameDT=off  OutDataTypeMode=boolean  OutDataTypeStr=boolean
  Multiport Switch : MultiPortSwitch  DataPortOrder=Zero-based contiguous  Inputs=4  zeroidx=on  OutDataType=sfix(16)  OutScaling=2^0
  Switch : Switch  Criteria=u2 ~= 0  OutDataType=sfix(16)  OutScaling=2^0
  Switch1 : Switch  Criteria=u2 ~= 0  OutDataType=sfix(16)  OutScaling=2^0
  Switch2 : Switch  Criteria=u2 ~= 0  OutDataType=sfix(16)  OutScaling=2^0
  Ready : Outport  OutDataType=sfix(16)  OutScaling=2^0
  wires:
  GBKind/1 -> Multiport Switch/1
  Multiport Switch/1 -> Logical Operator/1  "TransmOK"
  Brake/1 -> Compare To Constant/1
  Compare To Constant/1 -> Logical Operator/2
  Switch/1 -> Ready/1
  Logical Operator/1 -> Switch/2
  Constant1/1 -> Switch/3
  Constant/1 -> Switch/1
  Constant2/1 -> Multiport Switch/2
  Switch1/1 -> Multiport Switch/5, Multiport Switch/4
  Switch2/1 -> Multiport Switch/3
  Constant3/1 -> Switch2/3
  Constant4/1 -> Switch1/3
  Constant5/1 -> Switch2/1
  Constant6/1 -> Switch1/1
  Logical Operator1/1 -> Switch2/2
  Clutch/1 -> Compare To Constant1/1
  GearNoTrg/1 -> Compare To Zero/1
  Compare To Zero/1 -> Logical Operator1/1
  Compare To Constant1/1 -> Logical Operator1/2
  SelectorCtrl/1 -> Compare To Constant2/1
  Compare To Constant2/1 -> Switch1/2
